simulink model "uz_pmsm_model_6ph_dq"  (R2023a)
settings: Solver=FixedStepAuto  StartTime=0.0  StopTime=0.8  RelTol=1e-3
values from neighbouring files (symbols this model uses):
  c = 2/6*cat(1,tl1,tl2,tl3,tl4,tl5,tl6)    [uz_pmsm_model_6ph_dq_init_parameter.m]
  friction_coefficient = 0.001    [uz_pmsm_model_6ph_dq_init_parameter.m]
  inertia = 0.001    [uz_pmsm_model_6ph_dq_init_parameter.m]
  k_i_d = 50    [uz_pmsm_model_6ph_dq_init_parameter.m]
  k_i_q = 50    [uz_pmsm_model_6ph_dq_init_parameter.m]
  k_p_d = 0.5    [uz_pmsm_model_6ph_dq_init_parameter.m]
  k_p_q = 0.5    [uz_pmsm_model_6ph_dq_init_parameter.m]
  L_d = 0.46    [uz_pmsm_model_6ph_dq_init_parameter.m]
  L_q = 0.46    [uz_pmsm_model_6ph_dq_init_parameter.m]
  L_x = 0.08    [uz_pmsm_model_6ph_dq_init_parameter.m]
  L_y = 0.08    [uz_pmsm_model_6ph_dq_init_parameter.m]
  L_z1 = 0.08    [uz_pmsm_model_6ph_dq_init_parameter.m]
  L_z2 = 0.08    [uz_pmsm_model_6ph_dq_init_parameter.m]
  polepair = 3    [uz_pmsm_model_6ph_dq_init_parameter.m]
  psi_pm = 0.072    [uz_pmsm_model_6ph_dq_init_parameter.m]
  R_1 = 31.3    [uz_pmsm_model_6ph_dq_init_parameter.m]
  static_friction_torque = 0.001    [uz_pmsm_model_6ph_dq_init_parameter.m]
  ts_pmsm = 1e-6    (= 1e-06)    [uz_pmsm_model_6ph_dq_init_parameter.m]
undefined symbols (not defined in the file or in its folder): Kpd, Tnd
libraries: slpidlib x2, simulink x2, pid_lib x1, spsdq0toAlphaBetaZeroLib x1
settings Model: DataTypeOverride=Off  Creator=ts  LastModifiedBy=hufnagelde
settings SolverCC: AlgebraicLoopSolver=TrustRegion  AutoInsertRateTranBlk=on
settings DataIOCC: LimitDataPoints=on  SaveOutput=off  SaveTime=off
settings OptimizationCC: BlockReduction=off  ConditionallyExecuteInputs=off  DefaultParameterBehavior=Inlined  InheritOutputTypeSmallerThanSingle=on  LifeSpan=inf
settings DebuggingCC: AlgebraicLoopMsg=error  SingleTaskRateTransMsg=error  UnconnectedInputMsg=warning  UnconnectedOutputMsg=warning  UnconnectedLineMsg=warning  AllowSymbolicDim=off  StrictBusMsg=ErrorOnBusTreatedAsVector  SFUnexpectedBacktrackingDiag=warning  SFNoUnconditionalDefaultTransitionDiag=warning  SFExecutionAtInitializationDiag=none  ArithmeticOperatorsInVariantConditions=warning
settings HardwareCC: ProdBitPerPointer=32  ProdBitPerSizeT=32  ProdBitPerPtrDiffT=32  ProdLargestAtomicFloat=None  ProdIntDivRoundTo=Undefined  ProdEndianess=Unspecified  ProdWordSize=32  ProdHWDeviceType=ASIC/FPGA->ASIC/FPGA  ProdEqTarget=off
settings ModelReferenceCC: EnableRefExpFcnMdlSchedulingChecks=on
settings SFSimCC: SimUseLocalCustomCode=off  CustomCodeUndefinedFunction=UseInterfaceOnly
settings RTWCC: RTWUseLocalCustomCode=off  DLArmComputeVersion=19.05
settings CodeAppCC: StateflowObjectComments=on
settings GRTTargetCC: TargetLangStandard=C89/C90 (ANSI)
settings ConfigComp: CovScope=ReferencedModels  CovMetricSettings=dw  CovSaveCumulativeToWorkspaceVar=on  CovSaveSingleToWorkspaceVar=on  CovExternalEMLEnable=off  CovSFcnEnable=off

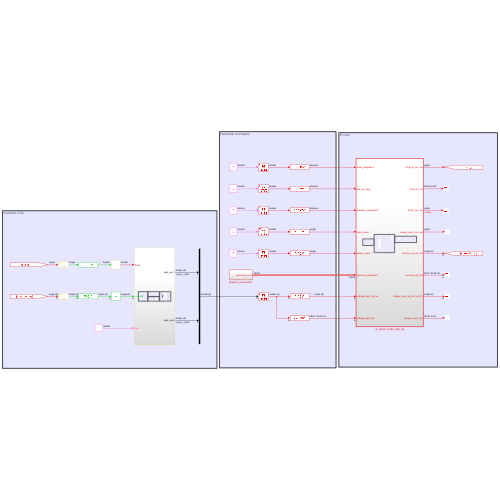
[thumbnail: Simulink's stored preview of the top-level diagram]
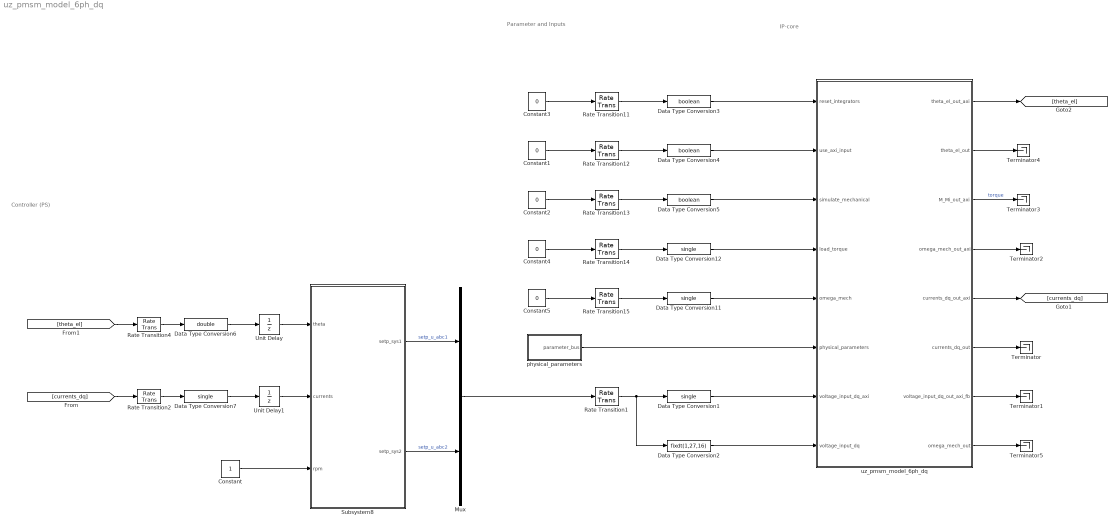
== system uz_pmsm_model_6ph_dq ==
  note: Controller (PS)
  note: Parameter and Inputs
  note: IP-core
  Constant : Constant
  Constant{1..5} (5 alike) : Constant  Value=0
  Data Type Conversion{1,7,11..12} (4 alike) : DataTypeConversion  OutDataTypeStr=single  SaturateOnIntegerOverflow=off  RndMeth=Floor
  Data Type Conversion2 : DataTypeConversion  OutDataTypeStr=fixdt(1,27,16)  SaturateOnIntegerOverflow=off  RndMeth=Floor
  Data Type Conversion3 : DataTypeConversion  OutDataTypeStr=boolean  SaturateOnIntegerOverflow=off  RndMeth=Floor
  Data Type Conversion4 : DataTypeConversion  OutDataTypeStr=boolean  SaturateOnIntegerOverflow=off  RndMeth=Floor
  Data Type Conversion5 : DataTypeConversion  OutDataTypeStr=boolean  SaturateOnIntegerOverflow=off  RndMeth=Floor
  Data Type Conversion6 : DataTypeConversion  OutDataTypeStr=double  SaturateOnIntegerOverflow=off  RndMeth=Floor
  Mux : Mux  Inputs=2
  Rate Transition{1,11..15} (6 alike) : RateTransition  OutPortSampleTime=ts_pmsm
  Rate Transition2 : RateTransition  OutPortSampleTime=ts_isr
  Rate Transition4 : RateTransition  OutPortSampleTime=ts_isr
  Subsystem8 : Subsystem
  Terminator{,1..5} (6 alike) : Terminator
  Unit Delay : UnitDelay  SampleTime=-1  HasFrameUpgradeWarning=on
  Unit Delay1 : UnitDelay  SampleTime=-1  HasFrameUpgradeWarning=on
  physical_parameters : Subsystem
  uz_pmsm_model_6ph_dq : Subsystem  TreatAsAtomicUnit=on
  wires:
  [theta_el] -> Rate Transition4/1
  Data Type Conversion6/1 -> Unit Delay/1
  Rate Transition4/1 -> Data Type Conversion6/1
  Constant3/1 -> Rate Transition11/1
  Rate Transition11/1 -> Data Type Conversion3/1
  Data Type Conversion3/1 -> uz_pmsm_model_6ph_dq/1(reset_integrators)
  Data Type Conversion4/1 -> uz_pmsm_model_6ph_dq/2(use_axi_input)
  Rate Transition12/1 -> Data Type Conversion4/1
  Constant1/1 -> Rate Transition12/1
  Constant2/1 -> Rate Transition13/1
  Rate Transition13/1 -> Data Type Conversion5/1
  Data Type Conversion5/1 -> uz_pmsm_model_6ph_dq/3(simulate_mechanical)
  Rate Transition15/1 -> Data Type Conversion11/1
  Rate Transition14/1 -> Data Type Conversion12/1
  Data Type Conversion12/1 -> uz_pmsm_model_6ph_dq/4(load_torque)
  Data Type Conversion11/1 -> uz_pmsm_model_6ph_dq/5(omega_mech)
  Constant5/1 -> Rate Transition15/1
  Constant4/1 -> Rate Transition14/1
  physical_parameters/1(parameter_bus) -> uz_pmsm_model_6ph_dq/6(physical_parameters)
  Subsystem8/2(setp_sys2) -> Mux/2  "setp_u_abc2"
  Subsystem8/1(setp_sys1) -> Mux/1  "setp_u_abc1"
  Rate Transition1/1 -> Data Type Conversion2/1, Data Type Conversion1/1
  Data Type Conversion1/1 -> uz_pmsm_model_6ph_dq/7(voltage_input_dq_axi)
  Data Type Conversion2/1 -> uz_pmsm_model_6ph_dq/8(voltage_input_dq)
  Mux/1 -> Rate Transition1/1
  Unit Delay/1 -> Subsystem8/1(theta)
  Unit Delay1/1 -> Subsystem8/2(currents)
  Rate Transition2/1 -> Data Type Conversion7/1
  Data Type Conversion7/1 -> Unit Delay1/1
  [currents_dq] -> Rate Transition2/1
  uz_pmsm_model_6ph_dq/1(theta_el_out_axi) -> [theta_el]
  uz_pmsm_model_6ph_dq/5(currents_dq_out_axi) -> [currents_dq]
  uz_pmsm_model_6ph_dq/6(currents_dq_out) -> Terminator/1
  uz_pmsm_model_6ph_dq/7(voltage_input_dq_out_axi_fb) -> Terminator1/1
  uz_pmsm_model_6ph_dq/4(omega_mech_out_axi) -> Terminator2/1
  uz_pmsm_model_6ph_dq/3(M_Mi_out_axi) -> Terminator3/1  "torque"
  uz_pmsm_model_6ph_dq/2(theta_el_out) -> Terminator4/1
  Constant/1 -> Subsystem8/3(rpm)
  uz_pmsm_model_6ph_dq/8(omega_mech_out) -> Terminator5/1

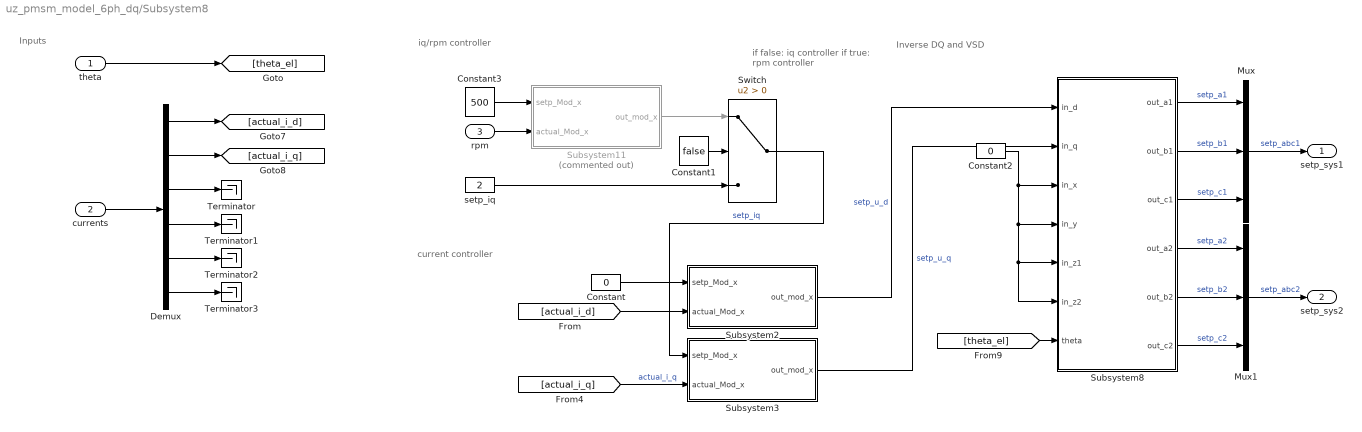
== system uz_pmsm_model_6ph_dq/Subsystem8 ==
  note: Inputs
  note: current controller
  note: iq/rpm controller
  note: if false: iq controller
      | if true: rpm controller
  note: Inverse DQ and VSD
  theta : Inport
  currents : Inport  Port=2
  rpm : Inport  Port=3
  Constant : Constant  Value=0
  Constant1 : Constant  Value=false
  Constant2 : Constant  Value=0
  Constant3 : Constant  Value=500
  Demux : Demux  Outputs=6
  Mux : Mux  Inputs=3
  Mux1 : Mux  Inputs=3
  Subsystem11 : Subsystem  Commented=on
  Subsystem2 : Subsystem
  Subsystem3 : Subsystem
  Subsystem8 : Subsystem
  Switch : Switch  Criteria=u2 > Threshold  SaturateOnIntegerOverflow=off  InputSameDT=off
  Terminator{,1..3} (4 alike) : Terminator
  setp_iq : Constant  Value=2
  setp_sys1 : Outport
  setp_sys2 : Outport  Port=2
  wires:
  Subsystem8/1(out_a1) -> Mux/1  "setp_a1"
  [theta_el] -> Subsystem8/7(theta)
  Subsystem8/2(out_b1) -> Mux/2  "setp_b1"
  Subsystem8/3(out_c1) -> Mux/3  "setp_c1"
  [actual_i_d] -> Subsystem2/2(actual_Mod_x)
  Constant/1 -> Subsystem2/1(setp_Mod_x)
  [actual_i_q] -> Subsystem3/2(actual_Mod_x)  "actual_i_q"
  theta/1 -> [theta_el]
  Mux/1 -> setp_sys1/1  "setp_abc1"
  Mux1/1 -> setp_sys2/1  "setp_abc2"
  Subsystem8/6(out_c2) -> Mux1/3  "setp_c2"
  Subsystem8/5(out_b2) -> Mux1/2  "setp_b2"
  Subsystem8/4(out_a2) -> Mux1/1  "setp_a2"
  rpm/1 -> Subsystem11/2(actual_Mod_x)
  Constant2/1 -> Subsystem8/3(in_x), Subsystem8/4(in_y), Subsystem8/5(in_z1), Subsystem8/6(in_z2)
  Subsystem11/1(out_mod_x) -> Switch/1
  Switch/1 -> Subsystem3/1(setp_Mod_x)  "setp_iq"
  Constant1/1 -> Switch/2
  setp_iq/1 -> Switch/3
  Constant3/1 -> Subsystem11/1(setp_Mod_x)
  Subsystem3/1(out_mod_x) -> Subsystem8/2(in_q)  "setp_u_q"
  Subsystem2/1(out_mod_x) -> Subsystem8/1(in_d)  "setp_u_d"
  currents/1 -> Demux/1
  Demux/1 -> [actual_i_d]
  Demux/2 -> [actual_i_q]
  Demux/3 -> Terminator/1
  Demux/4 -> Terminator1/1
  Demux/5 -> Terminator2/1
  Demux/6 -> Terminator3/1

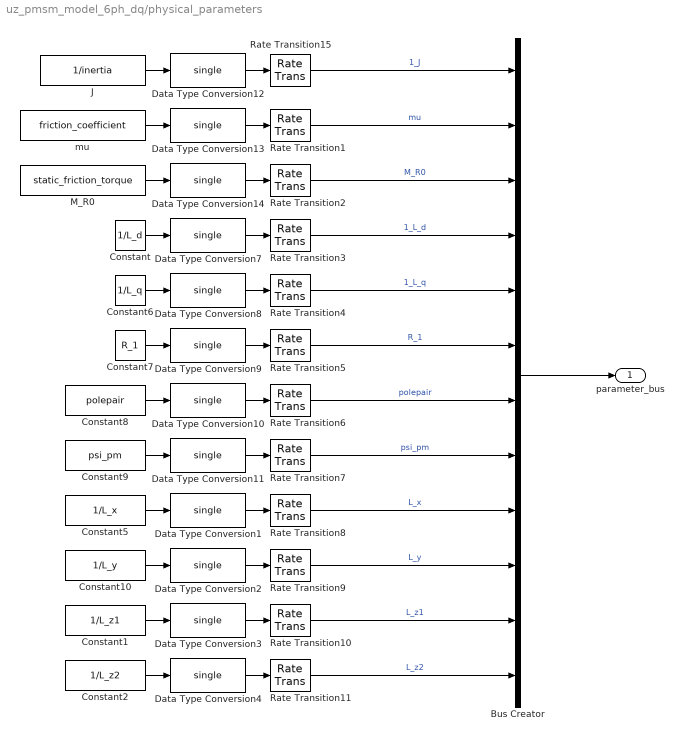
== system uz_pmsm_model_6ph_dq/physical_parameters ==
  Bus Creator : BusCreator  Inputs=12
  Constant : Constant  Value=1/L_d
  Constant1 : Constant  Value=1/L_z1
  Constant10 : Constant  Value=1/L_y
  Constant2 : Constant  Value=1/L_z2
  Constant5 : Constant  Value=1/L_x
  Constant6 : Constant  Value=1/L_q
  Constant7 : Constant  Value=R_1
  Constant8 : Constant  Value=polepair
  Constant9 : Constant  Value=psi_pm
  Data Type Conversion{1..4,7..14} (12 alike) : DataTypeConversion  OutDataTypeStr=single  SaturateOnIntegerOverflow=off  RndMeth=Floor
  J : Constant  Value=1/inertia
  M_R0 : Constant  Value=static_friction_torque
  Rate Transition{1..11,15} (12 alike) : RateTransition  OutPortSampleTime=ts_pmsm
  mu : Constant  Value=friction_coefficient
  parameter_bus : Outport
  wires:
  Data Type Conversion12/1 -> Rate Transition15/1
  Data Type Conversion7/1 -> Rate Transition3/1
  Rate Transition2/1 -> Bus Creator/3  "M_R0"
  Rate Transition7/1 -> Bus Creator/8  "psi_pm"
  Data Type Conversion14/1 -> Rate Transition2/1
  Rate Transition5/1 -> Bus Creator/6  "R_1"
  Rate Transition15/1 -> Bus Creator/1  "1_J"
  Rate Transition6/1 -> Bus Creator/7  "polepair"
  Bus Creator/1 -> parameter_bus/1
  Data Type Conversion11/1 -> Rate Transition7/1
  Constant8/1 -> Data Type Conversion10/1
  Data Type Conversion9/1 -> Rate Transition5/1
  Rate Transition1/1 -> Bus Creator/2  "mu"
  Constant6/1 -> Data Type Conversion8/1
  Rate Transition3/1 -> Bus Creator/4  "1_L_d"
  J/1 -> Data Type Conversion12/1
  Data Type Conversion8/1 -> Rate Transition4/1
  Data Type Conversion10/1 -> Rate Transition6/1
  mu/1 -> Data Type Conversion13/1
  M_R0/1 -> Data Type Conversion14/1
  Rate Transition4/1 -> Bus Creator/5  "1_L_q"
  Data Type Conversion13/1 -> Rate Transition1/1
  Constant7/1 -> Data Type Conversion9/1
  Constant9/1 -> Data Type Conversion11/1
  Constant/1 -> Data Type Conversion7/1
  Data Type Conversion1/1 -> Rate Transition8/1
  Data Type Conversion2/1 -> Rate Transition9/1
  Data Type Conversion3/1 -> Rate Transition10/1
  Data Type Conversion4/1 -> Rate Transition11/1
  Rate Transition8/1 -> Bus Creator/9  "L_x"
  Rate Transition11/1 -> Bus Creator/12  "L_z2"
  Rate Transition10/1 -> Bus Creator/11  "L_z1"
  Rate Transition9/1 -> Bus Creator/10  "L_y"
  Constant2/1 -> Data Type Conversion4/1
  Constant1/1 -> Data Type Conversion3/1
  Constant5/1 -> Data Type Conversion1/1
  Constant10/1 -> Data Type Conversion2/1

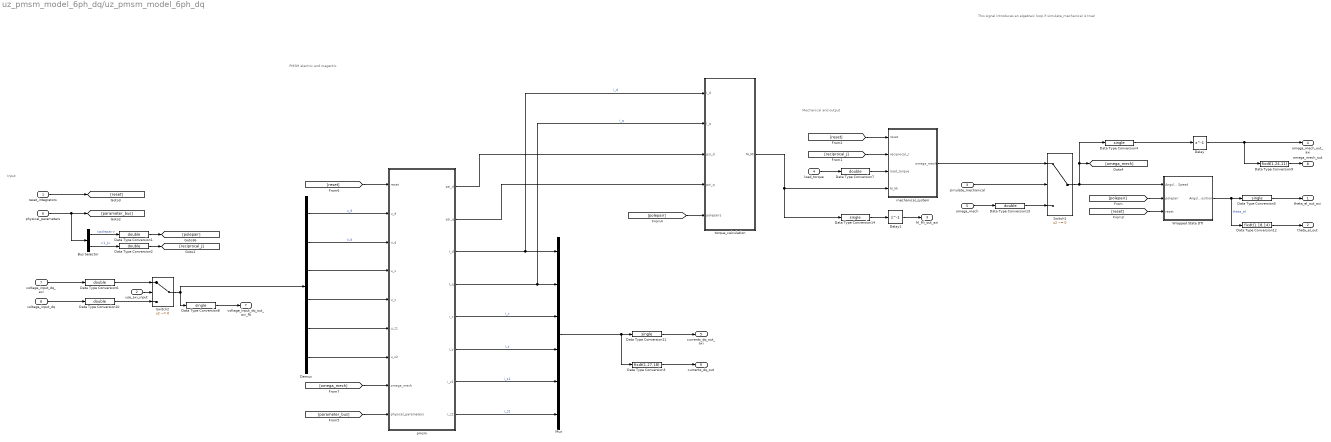
== system uz_pmsm_model_6ph_dq/uz_pmsm_model_6ph_dq ==
  note: Input
  note: This signal introduces an algebraic loop if simulate_mechanical is true!
  note: PMSM electric and magentic
  note: Mechanical and output
  reset_integrators : Inport
  use_axi_input : Inport  Port=2
  simulate_mechanical : Inport  Port=3
  load_torque : Inport  Port=4
  omega_mech : Inport  Port=5
  physical_parameters : Inport  Port=6
  voltage_input_dq_axi : Inport  Port=7
  voltage_input_dq : Inport  Port=8
  Bus Selector : BusSelector  OutputSignals=polepair,1_J
  Data Type Conversion{1..2,6..7,10,13} (6 alike) : DataTypeConversion  OutDataTypeStr=double  RndMeth=Nearest  SaturateOnIntegerOverflow=off
  Data Type Conversion{4..5,8,11,14} (5 alike) : DataTypeConversion  OutDataTypeStr=single  RndMeth=Nearest  SaturateOnIntegerOverflow=off
  Data Type Conversion12 : DataTypeConversion  OutDataTypeStr=fixdt(1,18,14)  RndMeth=Nearest  SaturateOnIntegerOverflow=off
  Data Type Conversion3 : DataTypeConversion  OutDataTypeStr=fixdt(1,27,18)  RndMeth=Nearest  SaturateOnIntegerOverflow=off
  Data Type Conversion9 : DataTypeConversion  OutDataTypeStr=fixdt(1,24,11)  RndMeth=Nearest  SaturateOnIntegerOverflow=off
  Delay : Delay  DelayLength=1
  Delay1 : Delay  DelayLength=1
  Demux : Demux  Outputs=6
  Mux : Mux  Inputs=6
  Switch1 : Switch  Criteria=u2 ~= 0  SaturateOnIntegerOverflow=off  InputSameDT=off
  Switch2 : Switch  Criteria=u2 ~= 0  SaturateOnIntegerOverflow=off  InputSameDT=off
  Wrapped State DTI : Subsystem
  mechanical_system : Subsystem
  pmsm : Subsystem
  torque_calculation : Subsystem
  theta_el_out_axi : Outport
  theta_el_out : Outport  Port=2
  M_Mi_out_axi : Outport  Port=3
  omega_mech_out_axi : Outport  Port=4
  currents_dq_out_axi : Outport  Port=5
  currents_dq_out : Outport  Port=6
  voltage_input_dq_out_axi_fb : Outport  Port=7
  omega_mech_out : Outport  Port=8
  wires:
  Demux/5 -> pmsm/6(u_z1)
  Demux/3 -> pmsm/4(u_x)
  pmsm/3(I_d) -> torque_calculation/1(I_d), Mux/1  "i_d"
  Demux/1 -> pmsm/2(u_d)  "u_d"
  pmsm/6(i_y) -> Mux/4  "i_y"
  Demux/4 -> pmsm/5(u_y)
  Demux/2 -> pmsm/3(u_q)  "u_q"
  pmsm/7(i_z1) -> Mux/5  "i_z1"
  torque_calculation/1(M_Mi) -> mechanical_system/4(M_Mi), Data Type Conversion14/1
  pmsm/1(psi_d) -> torque_calculation/3(psi_d)
  omega_mech/1 -> Data Type Conversion13/1
  pmsm/2(psi_q) -> torque_calculation/4(psi_q)
  simulate_mechanical/1 -> Switch1/2
  Demux/6 -> pmsm/7(u_z2)
  pmsm/5(i_x) -> Mux/3  "i_x"
  pmsm/4(I_q) -> torque_calculation/2(I_q), Mux/2  "i_q"
  mechanical_system/1(omega_mech) -> Switch1/1
  load_torque/1 -> Data Type Conversion7/1
  pmsm/8(i_z2) -> Mux/6  "i_z2"
  Mux/1 -> Data Type Conversion3/1, Data Type Conversion11/1
  Delay/1 -> Data Type Conversion9/1, omega_mech_out_axi/1
  Delay1/1 -> M_Mi_out_axi/1
  Switch2/1 -> Data Type Conversion8/1, Demux/1
  Data Type Conversion11/1 -> currents_dq_out_axi/1
  Data Type Conversion14/1 -> Delay1/1
  Data Type Conversion4/1 -> Delay/1
  Data Type Conversion5/1 -> theta_el_out_axi/1
  Wrapped State DTI/1(Angular Position) -> Data Type Conversion12/1, Data Type Conversion5/1  "theta_el"
  Data Type Conversion7/1 -> mechanical_system/3(load_torque)
  Data Type Conversion12/1 -> theta_el_out/1
  use_axi_input/1 -> Switch2/2
  voltage_input_dq/1 -> Data Type Conversion10/1
  voltage_input_dq_axi/1 -> Data Type Conversion6/1
  Data Type Conversion6/1 -> Switch2/1
  Data Type Conversion10/1 -> Switch2/3
  Data Type Conversion13/1 -> Switch1/3
  Data Type Conversion3/1 -> currents_dq_out/1
  [reciprocal_J] -> mechanical_system/2(reciprocal_J)
  [reset] -> mechanical_system/1(reset)
  [reset] -> Wrapped State DTI/3(reset)
  [polepair] -> Wrapped State DTI/2(polepair)
  [polepair] -> torque_calculation/5(polepairs)
  Data Type Conversion8/1 -> voltage_input_dq_out_axi_fb/1
  physical_parameters/1 -> Bus Selector/1, [parameter_bus]
  reset_integrators/1 -> [reset]
  [parameter_bus] -> pmsm/9(physical_parameters)
  Bus Selector/2 -> Data Type Conversion2/1  "<1_J>"
  Data Type Conversion1/1 -> [polepair]
  Bus Selector/1 -> Data Type Conversion1/1  "<polepair>"
  Data Type Conversion2/1 -> [reciprocal_J]
  Switch1/1 -> Data Type Conversion4/1, [omega_mech], Wrapped State DTI/1(Angular Speed)
  [omega_mech] -> pmsm/8(omega_mech)
  [reset] -> pmsm/1(reset)
  Data Type Conversion9/1 -> omega_mech_out/1

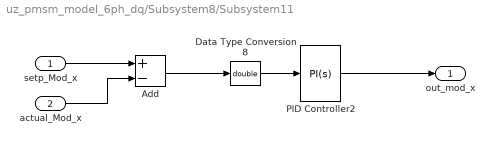
== system uz_pmsm_model_6ph_dq/Subsystem8/Subsystem11 ==
  setp_Mod_x : Inport
  actual_Mod_x : Inport  Port=2
  Add : Sum  Inputs=+-
  Data Type Conversion8 : DataTypeConversion  OutDataTypeStr=double  SaturateOnIntegerOverflow=off  RndMeth=Floor
  PID Controller2 : pid_lib/PID Controller  Controller=PI  Form=Ideal  TimeDomain=Continuous-time  UseExternalTs=off  SampleTime=-1  IntegratorMethod=Forward Euler  FilterMethod=Forward Euler  ControllerParametersSource=internal  P=Kpd  I=1/Tnd  D=0  N=100  UseFilter=on  TunerSelectOption=Transfer Function Based (PID Tuner App)  InitialConditionSource=internal  InitialConditionForIntegrator=0  InitialConditionForFilter=0  DifferentiatorICPrevScaledInput=0  ExternalReset=none  TrackingMode=off  Kt=1  LimitOutput=on  SatLimitsSource=internal  UpperSaturationLimit=50  LowerSaturationLimit=-50  LinearizeAsGain=on  AntiWindupMode=clamping  Kb=1  POutMin=[]  POutMax=[]  IOutMin=[]  IOutMax=[]  DOutMin=[]  DOutMax=[]  NOutMin=[]  NOutMax=[]  SumOutMin=[]  SumOutMax=[]  SaturationOutMin=[]  SaturationOutMax=[]  PParamMin=[]  PParamMax=[]  IParamMin=[]  IParamMax=[]  DParamMin=[]  DParamMax=[]  NParamMin=[]  NParamMax=[]  KbParamMin=[]  KbParamMax=[]  KtParamMin=[]  KtParamMax=[]  KbOutMin=[]  KbOutMax=[]  KtOutMin=[]  KtOutMax=[]  IntegratorOutMin=[]  IntegratorOutMax=[]  FilterOutMin=[]  FilterOutMax=[]  SumI1OutMin=[]  SumI1OutMax=[]  SumI2OutMin=[]  SumI2OutMax=[]  SumI3OutMin=[]  SumI3OutMax=[]  SumI4OutMin=[]  SumI4OutMax=[]  SumDOutMin=[]  SumDOutMax=[]  DifferentiatorOutMin=[]  DifferentiatorOutMax=[]  FilterDiffOutCoefMin=[]  FilterDiffOutCoefMax=[]  ReciprocalOutMin=[]  ReciprocalOutMax=[]  SumDenOutMin=[]  SumDenOutMax=[]  SumNumOutMin=[]  SumNumOutMax=[]  DivideOutMin=[]  DivideOutMax=[]  UdiffTsProdOutMin=[]  UdiffTsProdOutMax=[]  NTsProdOutMin=[]  NTsProdOutMax=[]  UintegralTsProdOutMin=[]  UintegralTsProdOutMax=[]  UngainTsProdOutMin=[]  UngainTsProdOutMax=[]  IntegratorContinuousStateAttributes=''  IntegratorStateMustResolveToSignalObject=off  IntegratorRTWStateStorageClass=Auto  FilterContinuousStateAttributes=''  FilterStateMustResolveToSignalObject=off  FilterRTWStateStorageClass=Auto  ParallelPVariant=Passthrough  IdealPVariant=InternalParameters  IVariant=InternalParameters  DVariant=Disabled  IntegratorVariant=Continuous  SatVariant=Enabled  AWVariant=ContClampingIdeal  PCopyVariant=InternalParamsIdeal  TRVariant=Disabled  FdbkBlocksVariant=Forward  IdealPFdbkVariant=Disabled  SatFdbkVariant=Disabled  DerivativeFilterVariant=Disabled  NVariant=Disabled  NCopyVariant=Disabled_SignalSpec  FilterICVariant=Disabled  IntegratorICVariant=InternalICs  ExternalResetVariant=Disabled  TRSumVariant=Passthrough  SumFdbkVariant=Disabled  SumVariant=Sum_PI  TsampFilterVariant=InternalTs  TsampNgainVariant=Passthrough  TsampIntegralVariant=Passthrough  ExternalSaturationOutDataTypeStr=Inherit: Same as second input
  out_mod_x : Outport
  wires:
  Add/1 -> Data Type Conversion8/1
  actual_Mod_x/1 -> Add/2
  Data Type Conversion8/1 -> PID Controller2/1
  setp_Mod_x/1 -> Add/1
  PID Controller2/1 -> out_mod_x/1

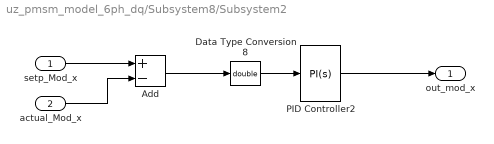
== system uz_pmsm_model_6ph_dq/Subsystem8/Subsystem2 ==
  setp_Mod_x : Inport
  actual_Mod_x : Inport  Port=2
  Add : Sum  Inputs=+-
  Data Type Conversion8 : DataTypeConversion  OutDataTypeStr=double  SaturateOnIntegerOverflow=off  RndMeth=Floor
  PID Controller2 : slpidlib/PID Controller  Controller=PI  Form=Ideal  TimeDomain=Continuous-time  UseExternalTs=off  SampleTime=-1  IntegratorMethod=Forward Euler  FilterMethod=Forward Euler  ControllerParametersSource=internal  P=k_p_d  I=k_i_d  UseKiTs=off  D=0  N=100  UseFilter=on  TunerSelectOption=Transfer Function Based (PID Tuner App)  InitialConditionSource=internal  InitialConditionForIntegrator=0  InitialConditionForFilter=0  DifferentiatorICPrevScaledInput=0  ExternalReset=none  TrackingMode=off  Kt=1  LimitOutput=on  SatLimitsSource=internal  UpperSaturationLimit=100  LowerSaturationLimit=-100  LinearizeAsGain=on  AntiWindupMode=clamping  Kb=1  LimitIntegrator=off  UpperIntegratorSaturationLimit=inf  LowerIntegratorSaturationLimit=-inf  POutMin=[]  POutMax=[]  IOutMin=[]  IOutMax=[]  DOutMin=[]  DOutMax=[]  NOutMin=[]  NOutMax=[]  SumOutMin=[]  SumOutMax=[]  SaturationOutMin=[]  SaturationOutMax=[]  PParamMin=[]  PParamMax=[]  IParamMin=[]  IParamMax=[]  DParamMin=[]  DParamMax=[]  NParamMin=[]  NParamMax=[]  KbParamMin=[]  KbParamMax=[]  KtParamMin=[]  KtParamMax=[]  KbOutMin=[]  KbOutMax=[]  KtOutMin=[]  KtOutMax=[]  IntegratorOutMin=[]  IntegratorOutMax=[]  FilterOutMin=[]  FilterOutMax=[]  SumI1OutMin=[]  SumI1OutMax=[]  SumI2OutMin=[]  SumI2OutMax=[]  SumI3OutMin=[]  SumI3OutMax=[]  SumI4OutMin=[]  SumI4OutMax=[]  SumDOutMin=[]  SumDOutMax=[]  DifferentiatorOutMin=[]  DifferentiatorOutMax=[]  FilterDiffOutCoefMin=[]  FilterDiffOutCoefMax=[]  ReciprocalOutMin=[]  ReciprocalOutMax=[]  SumDenOutMin=[]  SumDenOutMax=[]  SumNumOutMin=[]  SumNumOutMax=[]  DivideOutMin=[]  DivideOutMax=[]  UdiffTsProdOutMin=[]  UdiffTsProdOutMax=[]  NTsProdOutMin=[]  NTsProdOutMax=[]  UintegralTsProdOutMin=[]  UintegralTsProdOutMax=[]  UngainTsProdOutMin=[]  UngainTsProdOutMax=[]  ClampingZeroOutDataTypeStr=Inherit: Inherit via back propagation  ClampingZeroOutMin=[]  ClampingZeroOutMax=[]  FilterDenConstantOutDataTypeStr=Inherit: Inherit via back propagation  FilterDenConstantOutMin=[]  FilterDenConstantOutMax=[]  PCopyOutDataTypeStr=Inherit: Inherit via back propagation  PCopyOutMin=[]  PCopyOutMax=[]  NCopyOutDataTypeStr=Inherit: Inherit via back propagation  NCopyOutMin=[]  NCopyOutMax=[]  IntegratorContinuousStateAttributes=''  IntegratorStateMustResolveToSignalObject=off  IntegratorRTWStateStorageClass=Auto  FilterContinuousStateAttributes=''  FilterStateMustResolveToSignalObject=off  FilterRTWStateStorageClass=Auto  ParallelPVariant=Passthrough  IdealPVariant=InternalParameters  IVariant=InternalParameters  DVariant=Disabled  IntegratorVariant=Continuous  SatVariant=Enabled  AWVariant=ContClampingIdeal  PCopyVariant=InternalParamsIdeal  TRVariant=Disabled  FdbkBlocksVariant=Forward  IdealPFdbkVariant=Disabled  SatFdbkVariant=Disabled  DerivativeFilterVariant=Disabled  NVariant=Disabled  NCopyVariant=Disabled_SignalSpec  FilterICVariant=Disabled  IntegratorICVariant=InternalICs  ExternalResetVariant=Disabled  TRSumVariant=Passthrough  SumFdbkVariant=Disabled  SumVariant=Sum_PI  TsampFilterVariant=InternalTs  TsampNgainVariant=Passthrough  TsampIntegralVariant=Disabled_SignalSpec  ExternalSaturationOutDataTypeStr=Inherit: Same as second input
  out_mod_x : Outport
  wires:
  Add/1 -> Data Type Conversion8/1
  actual_Mod_x/1 -> Add/2
  Data Type Conversion8/1 -> PID Controller2/1
  setp_Mod_x/1 -> Add/1
  PID Controller2/1 -> out_mod_x/1

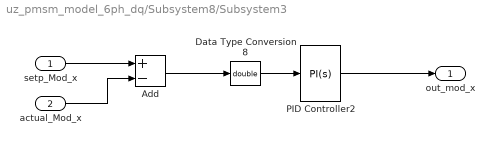
== system uz_pmsm_model_6ph_dq/Subsystem8/Subsystem3 ==
  setp_Mod_x : Inport
  actual_Mod_x : Inport  Port=2
  Add : Sum  Inputs=+-
  Data Type Conversion8 : DataTypeConversion  OutDataTypeStr=double  SaturateOnIntegerOverflow=off  RndMeth=Floor
  PID Controller2 : slpidlib/PID Controller  Controller=PI  Form=Ideal  TimeDomain=Continuous-time  UseExternalTs=off  SampleTime=-1  IntegratorMethod=Forward Euler  FilterMethod=Forward Euler  ControllerParametersSource=internal  P=k_p_q  I=k_i_q  UseKiTs=off  D=0  N=100  UseFilter=on  TunerSelectOption=Transfer Function Based (PID Tuner App)  InitialConditionSource=internal  InitialConditionForIntegrator=0  InitialConditionForFilter=0  DifferentiatorICPrevScaledInput=0  ExternalReset=none  TrackingMode=off  Kt=1  LimitOutput=on  SatLimitsSource=internal  UpperSaturationLimit=100  LowerSaturationLimit=-100  LinearizeAsGain=on  AntiWindupMode=clamping  Kb=1  LimitIntegrator=off  UpperIntegratorSaturationLimit=inf  LowerIntegratorSaturationLimit=-inf  POutMin=[]  POutMax=[]  IOutMin=[]  IOutMax=[]  DOutMin=[]  DOutMax=[]  NOutMin=[]  NOutMax=[]  SumOutMin=[]  SumOutMax=[]  SaturationOutMin=[]  SaturationOutMax=[]  PParamMin=[]  PParamMax=[]  IParamMin=[]  IParamMax=[]  DParamMin=[]  DParamMax=[]  NParamMin=[]  NParamMax=[]  KbParamMin=[]  KbParamMax=[]  KtParamMin=[]  KtParamMax=[]  KbOutMin=[]  KbOutMax=[]  KtOutMin=[]  KtOutMax=[]  IntegratorOutMin=[]  IntegratorOutMax=[]  FilterOutMin=[]  FilterOutMax=[]  SumI1OutMin=[]  SumI1OutMax=[]  SumI2OutMin=[]  SumI2OutMax=[]  SumI3OutMin=[]  SumI3OutMax=[]  SumI4OutMin=[]  SumI4OutMax=[]  SumDOutMin=[]  SumDOutMax=[]  DifferentiatorOutMin=[]  DifferentiatorOutMax=[]  FilterDiffOutCoefMin=[]  FilterDiffOutCoefMax=[]  ReciprocalOutMin=[]  ReciprocalOutMax=[]  SumDenOutMin=[]  SumDenOutMax=[]  SumNumOutMin=[]  SumNumOutMax=[]  DivideOutMin=[]  DivideOutMax=[]  UdiffTsProdOutMin=[]  UdiffTsProdOutMax=[]  NTsProdOutMin=[]  NTsProdOutMax=[]  UintegralTsProdOutMin=[]  UintegralTsProdOutMax=[]  UngainTsProdOutMin=[]  UngainTsProdOutMax=[]  ClampingZeroOutDataTypeStr=Inherit: Inherit via back propagation  ClampingZeroOutMin=[]  ClampingZeroOutMax=[]  FilterDenConstantOutDataTypeStr=Inherit: Inherit via back propagation  FilterDenConstantOutMin=[]  FilterDenConstantOutMax=[]  PCopyOutDataTypeStr=Inherit: Inherit via back propagation  PCopyOutMin=[]  PCopyOutMax=[]  NCopyOutDataTypeStr=Inherit: Inherit via back propagation  NCopyOutMin=[]  NCopyOutMax=[]  IntegratorContinuousStateAttributes=''  IntegratorStateMustResolveToSignalObject=off  IntegratorRTWStateStorageClass=Auto  FilterContinuousStateAttributes=''  FilterStateMustResolveToSignalObject=off  FilterRTWStateStorageClass=Auto  ParallelPVariant=Passthrough  IdealPVariant=InternalParameters  IVariant=InternalParameters  DVariant=Disabled  IntegratorVariant=Continuous  SatVariant=Enabled  AWVariant=ContClampingIdeal  PCopyVariant=InternalParamsIdeal  TRVariant=Disabled  FdbkBlocksVariant=Forward  IdealPFdbkVariant=Disabled  SatFdbkVariant=Disabled  DerivativeFilterVariant=Disabled  NVariant=Disabled  NCopyVariant=Disabled_SignalSpec  FilterICVariant=Disabled  IntegratorICVariant=InternalICs  ExternalResetVariant=Disabled  TRSumVariant=Passthrough  SumFdbkVariant=Disabled  SumVariant=Sum_PI  TsampFilterVariant=InternalTs  TsampNgainVariant=Passthrough  TsampIntegralVariant=Disabled_SignalSpec  ExternalSaturationOutDataTypeStr=Inherit: Same as second input
  out_mod_x : Outport
  wires:
  PID Controller2/1 -> out_mod_x/1
  setp_Mod_x/1 -> Add/1
  Data Type Conversion8/1 -> PID Controller2/1
  actual_Mod_x/1 -> Add/2
  Add/1 -> Data Type Conversion8/1

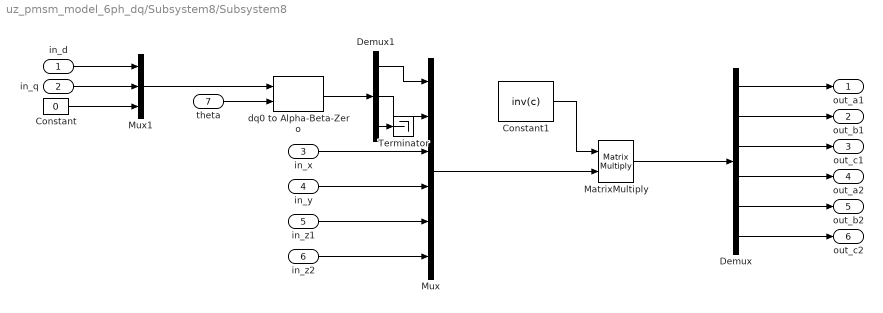
== system uz_pmsm_model_6ph_dq/Subsystem8/Subsystem8 ==
  in_d : Inport
  in_q : Inport  Port=2
  in_x : Inport  Port=3
  in_y : Inport  Port=4
  in_z1 : Inport  Port=5
  in_z2 : Inport  Port=6
  theta : Inport  Port=7
  Constant : Constant  Value=0  SampleTime=-1
  Constant1 : Constant  Value=inv(c)
  Demux : Demux  Outputs=6
  Demux1 : Demux  Outputs=3
  MatrixMultiply : Product  Multiplication=Matrix(*)
  Mux : Mux  Inputs=6
  Mux1 : Mux  Inputs=3
  Terminator : Terminator
  dq0 to Alpha-Beta-Zero : spsdq0toAlphaBetaZeroLib/dq0 to Alpha-Beta-Zero  Alignment=90 degrees behind phase A axis
  out_a1 : Outport
  out_b1 : Outport  Port=2
  out_c1 : Outport  Port=3
  out_a2 : Outport  Port=4
  out_b2 : Outport  Port=5
  out_c2 : Outport  Port=6
  wires:
  MatrixMultiply/1 -> Demux/1
  in_z2/1 -> Mux/6
  Demux/1 -> out_a1/1
  in_x/1 -> Mux/3
  in_y/1 -> Mux/4
  Mux/1 -> MatrixMultiply/2
  in_z1/1 -> Mux/5
  Constant/1 -> Mux1/3
  in_q/1 -> Mux1/2
  in_d/1 -> Mux1/1
  Mux1/1 -> dq0 to Alpha-Beta-Zero/1
  theta/1 -> dq0 to Alpha-Beta-Zero/2
  dq0 to Alpha-Beta-Zero/1 -> Demux1/1
  Demux1/1 -> Mux/1
  Demux1/2 -> Mux/2
  Demux1/3 -> Terminator/1
  Constant1/1 -> MatrixMultiply/1
  Demux/2 -> out_b1/1
  Demux/3 -> out_c1/1
  Demux/4 -> out_a2/1
  Demux/6 -> out_c2/1
  Demux/5 -> out_b2/1

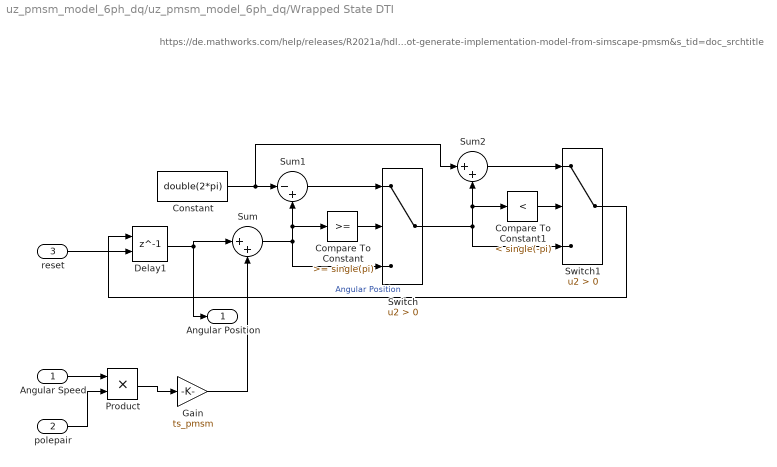
== system uz_pmsm_model_6ph_dq/uz_pmsm_model_6ph_dq/Wrapped State DTI ==
  note: https://de.mathworks.com/help/releases/R2021a/hdlcoder/ug/troubleshoot-generate-implementation-model-from-simscape-pmsm.html?searchHighlight=troubleshoot-generate-implementation-model-from-simscape-pmsm&s_tid=doc_srchtitle
  Angular Speed : Inport
  polepair : Inport  Port=2
  reset : Inport  Port=3
  Compare To Constant : simulink/Logic and Bit Operations/Compare To Constant  relop=>=  const=single(pi)  OutDataTypeStr=boolean
  Compare To Constant1 : simulink/Logic and Bit Operations/Compare To Constant  relop=<  const=single(-pi)  OutDataTypeStr=boolean
  Constant : Constant  Value=double(2*pi)  SampleTime=-1
  Delay1 : Delay  DelayLength=1  ExternalReset=Level
      settings: InputPortMap=u0,r5
  Gain : Gain  Gain=ts_pmsm
  Product : Product
  Sum : Sum  Inputs=|++
  Sum1 : Sum  Inputs=|-+
  Sum2 : Sum  Inputs=|++
  Switch : Switch  Criteria=u2 > Threshold  SaturateOnIntegerOverflow=off  InputSameDT=off
  Switch1 : Switch  Criteria=u2 > Threshold  SaturateOnIntegerOverflow=off  InputSameDT=off
  Angular Position : Outport
  wires:
  Compare To Constant1/1 -> Switch1/2
  Delay1/1 -> Sum/1, Angular Position/1
  Constant/1 -> Sum2/1, Sum1/1
  Sum2/1 -> Switch1/1
  Switch1/1 -> Delay1/1  "Angular Position"
  Switch/1 -> Sum2/2, Compare To Constant1/1, Switch1/3
  Compare To Constant/1 -> Switch/2
  Sum/1 -> Compare To Constant/1, Sum1/2, Switch/3
  Sum1/1 -> Switch/1
  Gain/1 -> Sum/2
  reset/1 -> Delay1/2
  Product/1 -> Gain/1
  Angular Speed/1 -> Product/1
  polepair/1 -> Product/2

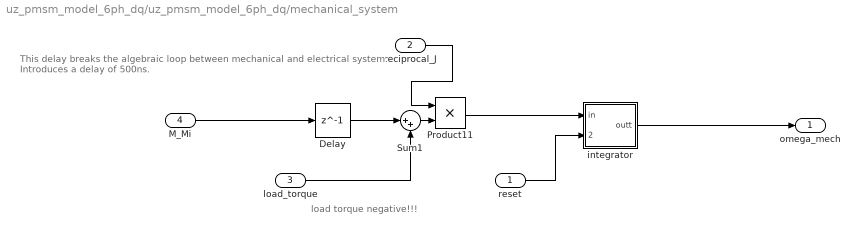
== system uz_pmsm_model_6ph_dq/uz_pmsm_model_6ph_dq/mechanical_system ==
  note: load torque negative!!!
  note: This delay breaks the algebraic loop between mechanical and electrical system.
      | Introduces a delay of 500ns.
  reset : Inport
  reciprocal_J : Inport  Port=2
  load_torque : Inport  Port=3
  M_Mi : Inport  Port=4
  Delay : Delay  DelayLength=1
  Product11 : Product
  Sum1 : Sum  Inputs=|++
  integrator : Subsystem
  omega_mech : Outport
  wires:
  reciprocal_J/1 -> Product11/1
  Sum1/1 -> Product11/2
  load_torque/1 -> Sum1/2
  M_Mi/1 -> Delay/1
  Delay/1 -> Sum1/1
  integrator/1(outt) -> omega_mech/1
  Product11/1 -> integrator/1(in)
  reset/1 -> integrator/2(reset)

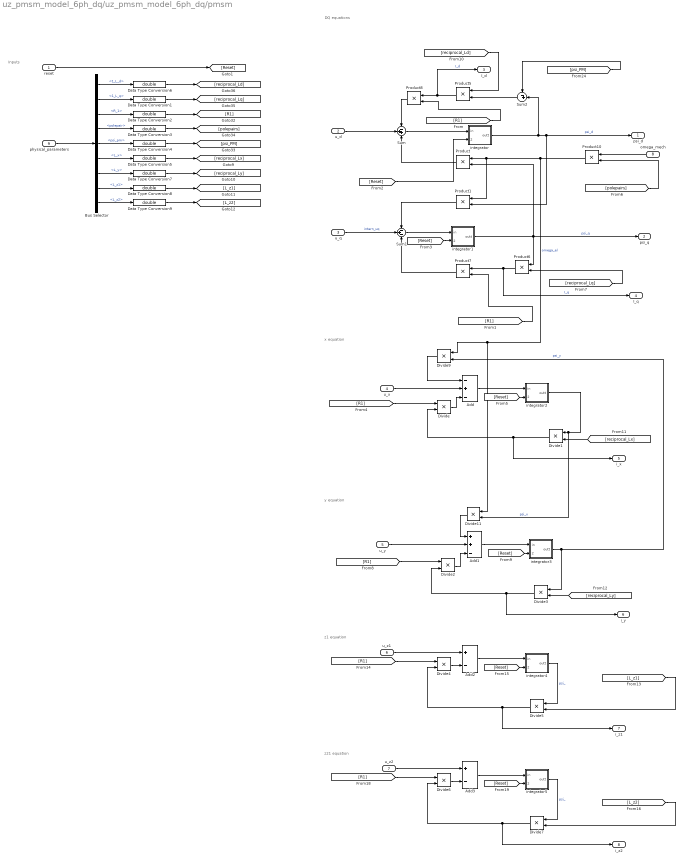
== system uz_pmsm_model_6ph_dq/uz_pmsm_model_6ph_dq/pmsm ==
  note: Inputs
  note: x equation
  note: DQ equations
  note: y equation
  note: z1 equation
  note: z21 equation
  reset : Inport
  u_d : Inport  Port=2
  u_q : Inport  Port=3
  u_x : Inport  Port=4
  u_y : Inport  Port=5
  u_z1 : Inport  Port=6
  u_z2 : Inport  Port=7
  omega_mech : Inport  Port=8
  physical_parameters : Inport  Port=9
  Add : Sum  Inputs=-+-
  Add1 : Sum  Inputs=++-
  Add2 : Sum  Inputs=+-
  Add3 : Sum  Inputs=+-
  Bus Selector : BusSelector  OutputSignals=1_L_d,1_L_q,R_1,polepair,psi_pm,L_x,L_y,L_z1,L_z2
  Data Type Conversion{1..9} (9 alike) : DataTypeConversion  OutDataTypeStr=double  RndMeth=Nearest  SaturateOnIntegerOverflow=off
  Divide{,1..7,9,11} (10 alike) : Product  Inputs=**
  Product{,1,5..8,10} (7 alike) : Product
  Sum : Sum  Inputs=-++
  Sum1 : Sum  Inputs=-+-
  Sum2 : Sum  Inputs=-+|
  integrator : Subsystem
  integrator1 : Subsystem
  integrator2 : Subsystem
  integrator3 : Subsystem
  integrator4 : Subsystem
  integrator5 : Subsystem
  psi_d : Outport
  psi_q : Outport  Port=2
  I_d : Outport  Port=3
  I_q : Outport  Port=4
  i_x : Outport  Port=5
  i_y : Outport  Port=6
  i_z1 : Outport  Port=7
  i_z2 : Outport  Port=8
  wires:
  omega_mech/1 -> Product10/1
  u_q/1 -> Sum1/2  "intern_uq"
  Product/1 -> Sum/3
  Product5/1 -> I_d/1, Product8/1  "I_d"
  [reciprocal_Ld] -> Product5/1
  integrator1/1(outt) -> psi_q/1, Product/2, Product6/1  "psi_q"
  Product1/1 -> Sum1/1
  [psi_PM] -> Sum2/1
  Product6/1 -> I_q/1, Product7/1  "I_q"
  Product10/1 -> Divide9/1, Divide11/1, Product1/1, Product/1  "omega_el"
  integrator/1(outt) -> Sum2/2, psi_d/1, Product1/2  "psi_d"
  Sum2/1 -> Product5/2
  Product8/1 -> Sum/1
  [reciprocal_Lq] -> Product6/2
  Product7/1 -> Sum1/3
  reset/1 -> [Reset]
  [Reset] -> integrator/2(reset)
  [Reset] -> integrator1/2(reset)
  [Reset] -> integrator2/2(reset)
  [reciprocal_Lx] -> Divide1/2
  u_x/1 -> Add/2
  Divide1/1 -> Divide/2, i_x/1
  Divide/1 -> Add/3
  [R1] -> Divide/1
  integrator2/1(outt) -> Divide11/2, Divide1/1  "psi_x"
  integrator3/1(outt) -> Divide9/2, Divide3/1  "psi_y"
  [R1] -> Divide2/1
  Divide2/1 -> Add1/3
  Divide3/1 -> Divide2/2, i_y/1
  u_y/1 -> Add1/2
  [reciprocal_Ly] -> Divide3/2
  [Reset] -> integrator3/2(reset)
  [Reset] -> integrator4/2(reset)
  u_z1/1 -> Add2/1
  Divide5/1 -> i_z1/1, Divide4/2
  Divide4/1 -> Add2/2
  [R1] -> Divide4/1
  integrator4/1(outt) -> Divide5/1  "psi_"
  integrator5/1(outt) -> Divide7/1  "psi_"
  [R1] -> Divide6/1
  Divide6/1 -> Add3/2
  Divide7/1 -> i_z2/1, Divide6/2
  u_z2/1 -> Add3/1
  [Reset] -> integrator5/2(reset)
  physical_parameters/1 -> Bus Selector/1
  [polepairs] -> Product10/2
  [L_z1] -> Divide5/2
  [L_z2] -> Divide7/2
  Sum/1 -> integrator/1(in)
  Sum1/1 -> integrator1/1(in)
  Add/1 -> integrator2/1(in)
  Add1/1 -> integrator3/1(in)
  Add2/1 -> integrator4/1(in)
  Add3/1 -> integrator5/1(in)
  u_d/1 -> Sum/2
  Bus Selector/1 -> Data Type Conversion6/1  "<1_L_d>"
  Bus Selector/2 -> Data Type Conversion1/1  "<1_L_q>"
  Bus Selector/3 -> Data Type Conversion2/1  "<R_1>"
  Bus Selector/4 -> Data Type Conversion3/1  "<polepair>"
  Bus Selector/5 -> Data Type Conversion4/1  "<psi_pm>"
  Bus Selector/6 -> Data Type Conversion5/1  "<L_x>"
  Bus Selector/7 -> Data Type Conversion7/1  "<L_y>"
  Bus Selector/8 -> Data Type Conversion8/1  "<L_z1>"
  Bus Selector/9 -> Data Type Conversion9/1  "<L_z2>"
  Data Type Conversion9/1 -> [L_z2]
  Data Type Conversion8/1 -> [L_z1]
  Data Type Conversion7/1 -> [reciprocal_Ly]
  Data Type Conversion5/1 -> [reciprocal_Lx]
  Data Type Conversion4/1 -> [psi_PM]
  Data Type Conversion3/1 -> [polepairs]
  Data Type Conversion2/1 -> [R1]
  Data Type Conversion1/1 -> [reciprocal_Lq]
  Data Type Conversion6/1 -> [reciprocal_Ld]
  [R1] -> Product8/2
  [R1] -> Product7/2
  Divide9/1 -> Add/1
  Divide11/1 -> Add1/1

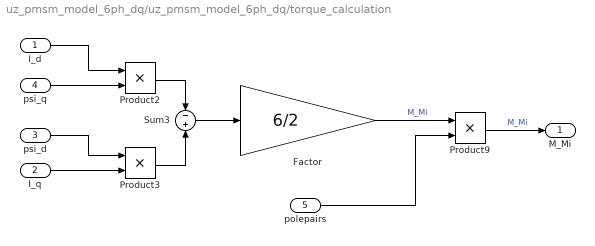
== system uz_pmsm_model_6ph_dq/uz_pmsm_model_6ph_dq/torque_calculation ==
  I_d : Inport
  I_q : Inport  Port=2
  psi_d : Inport  Port=3
  psi_q : Inport  Port=4
  polepairs : Inport  Port=5
  Factor : Gain  Gain=6/2
  Product2 : Product
  Product3 : Product
  Product9 : Product
  Sum3 : Sum  Inputs=-|+
  M_Mi : Outport
  wires:
  Sum3/1 -> Factor/1
  Product3/1 -> Sum3/2
  Product2/1 -> Sum3/1
  psi_q/1 -> Product2/2
  psi_d/1 -> Product3/1
  I_d/1 -> Product2/1
  I_q/1 -> Product3/2
  Product9/1 -> M_Mi/1  "M_Mi"
  polepairs/1 -> Product9/2
  Factor/1 -> Product9/1  "M_Mi"

== system uz_pmsm_model_6ph_dq/uz_pmsm_model_6ph_dq/mechanical_system/integrator ==
  in : Inport
  reset : Inport  Port=2
  Delay1 : Delay  DelayLength=1  ExternalReset=Level
      settings: InputPortMap=u0,r5
  Gain : Gain  Gain=ts_pmsm  OutDataTypeStr=Inherit: Same as input
  Sum3 : Sum  Inputs=|++  OutDataTypeStr=Inherit: Same as first input
  outt : Outport
  wires:
  reset/1 -> Delay1/2
  Gain/1 -> Sum3/1
  in/1 -> Gain/1
  Delay1/1 -> outt/1, Sum3/2
  Sum3/1 -> Delay1/1

== system uz_pmsm_model_6ph_dq/uz_pmsm_model_6ph_dq/pmsm/integrator ==
  in : Inport
  reset : Inport  Port=2
  Delay1 : Delay  DelayLength=1  ExternalReset=Level
      settings: InputPortMap=u0,r5
  Gain : Gain  Gain=ts_pmsm  OutDataTypeStr=Inherit: Same as input
  Sum3 : Sum  Inputs=|++  OutDataTypeStr=Inherit: Same as first input
  outt : Outport
  wires:
  reset/1 -> Delay1/2
  Gain/1 -> Sum3/1
  in/1 -> Gain/1
  Delay1/1 -> outt/1, Sum3/2
  Sum3/1 -> Delay1/1

== system uz_pmsm_model_6ph_dq/uz_pmsm_model_6ph_dq/pmsm/integrator1 ==
  in : Inport
  reset : Inport  Port=2
  Delay1 : Delay  DelayLength=1  ExternalReset=Level
      settings: InputPortMap=u0,r5
  Gain : Gain  Gain=ts_pmsm  OutDataTypeStr=Inherit: Same as input
  Sum3 : Sum  Inputs=|++  OutDataTypeStr=Inherit: Same as first input
  outt : Outport
  wires:
  reset/1 -> Delay1/2
  Gain/1 -> Sum3/1
  in/1 -> Gain/1
  Delay1/1 -> outt/1, Sum3/2
  Sum3/1 -> Delay1/1

== system uz_pmsm_model_6ph_dq/uz_pmsm_model_6ph_dq/pmsm/integrator2 ==
  in : Inport
  reset : Inport  Port=2
  Delay1 : Delay  DelayLength=1  ExternalReset=Level
      settings: InputPortMap=u0,r5
  Gain : Gain  Gain=ts_pmsm  OutDataTypeStr=Inherit: Same as input
  Sum3 : Sum  Inputs=|++  OutDataTypeStr=Inherit: Same as first input
  outt : Outport
  wires:
  reset/1 -> Delay1/2
  Gain/1 -> Sum3/1
  in/1 -> Gain/1
  Delay1/1 -> outt/1, Sum3/2
  Sum3/1 -> Delay1/1

== system uz_pmsm_model_6ph_dq/uz_pmsm_model_6ph_dq/pmsm/integrator3 ==
  in : Inport
  reset : Inport  Port=2
  Delay1 : Delay  DelayLength=1  ExternalReset=Level
      settings: InputPortMap=u0,r5
  Gain : Gain  Gain=ts_pmsm  OutDataTypeStr=Inherit: Same as input
  Sum3 : Sum  Inputs=|++  OutDataTypeStr=Inherit: Same as first input
  outt : Outport
  wires:
  Sum3/1 -> Delay1/1
  Delay1/1 -> Sum3/2, outt/1
  in/1 -> Gain/1
  Gain/1 -> Sum3/1
  reset/1 -> Delay1/2

== system uz_pmsm_model_6ph_dq/uz_pmsm_model_6ph_dq/pmsm/integrator4 ==
  in : Inport
  reset : Inport  Port=2
  Delay1 : Delay  DelayLength=1  ExternalReset=Level
      settings: InputPortMap=u0,r5
  Gain : Gain  Gain=ts_pmsm  OutDataTypeStr=Inherit: Same as input
  Sum3 : Sum  Inputs=|++  OutDataTypeStr=Inherit: Same as first input
  outt : Outport
  wires:
  reset/1 -> Delay1/2
  Gain/1 -> Sum3/1
  in/1 -> Gain/1
  Delay1/1 -> outt/1, Sum3/2
  Sum3/1 -> Delay1/1

== system uz_pmsm_model_6ph_dq/uz_pmsm_model_6ph_dq/pmsm/integrator5 ==
  in : Inport
  reset : Inport  Port=2
  Delay1 : Delay  DelayLength=1  ExternalReset=Level
      settings: InputPortMap=u0,r5
  Gain : Gain  Gain=ts_pmsm  OutDataTypeStr=Inherit: Same as input
  Sum3 : Sum  Inputs=|++  OutDataTypeStr=Inherit: Same as first input
  outt : Outport
  wires:
  Sum3/1 -> Delay1/1
  Delay1/1 -> Sum3/2, outt/1
  in/1 -> Gain/1
  Gain/1 -> Sum3/1
  reset/1 -> Delay1/2
